simulink model "sl_pmsm"  (R2023b)
settings: Solver=VariableStepAuto  StartTime=0.0  StopTime=1.0  RelTol=1e-3
InitFcn:
  | init
values from neighbouring files (symbols this model uses):
  pa = block.DialogPrm(1).Data    [current_controller.m]    (also in voltage_equation_dq.m)
libraries: spsVoltageMeasurementLib x9, spsSeriesRLCBranchLib x3, simulink x3, spsDCVoltageSourceLib x2, slpidlib x1, spsGroundLib x1, spsUniversalBridgeLib x1, spspowerguiLib x1
settings Model: Creator=PC  LastModifiedBy=PC

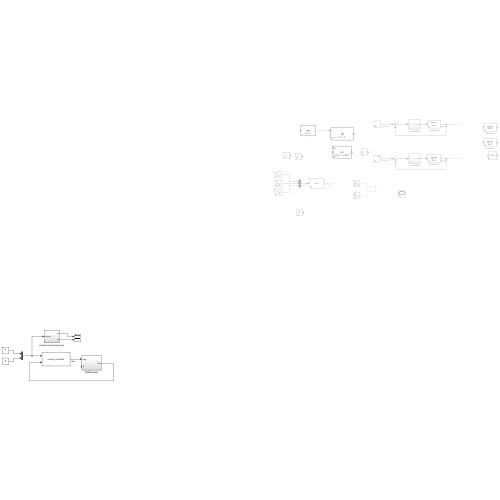
[thumbnail: Simulink's stored preview of the top-level diagram]
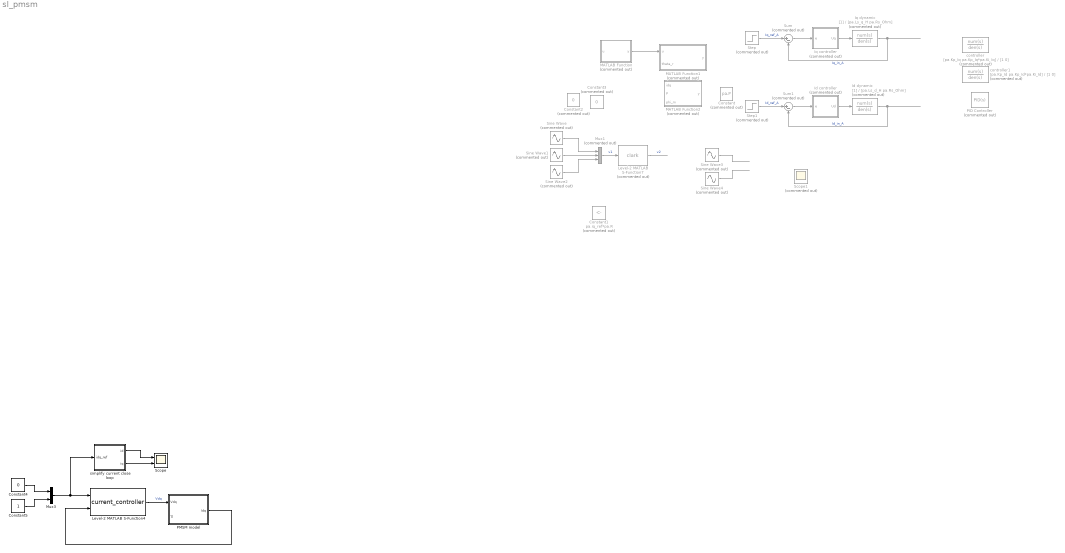
== system sl_pmsm ==
  Constant : Constant  Commented=on  Value=pa.P
  Constant1 : Constant  Commented=on  Value=pa.iq_ref*pa.R
  Constant2 : Constant  Commented=on  Value=0
  Constant3 : Constant  Commented=on  Value=0
  Constant4 : Constant  Value=0
  Constant5 : Constant
  Id controller : Subsystem  Commented=on
  Id dynamic : TransferFcn  Commented=on  Denominator=[pa.Ls_d_H pa.Rs_Ohm]
  Iq controller : Subsystem  Commented=on
  Iq dynamic : TransferFcn  Commented=on  Denominator=[pa.Ls_q_H pa.Rs_Ohm]
  Level-2 MATLAB S-Function4 : M-S-Function  FunctionName=current_controller  Parameters=pa
  Level-2 MATLAB S-Function7 : M-S-Function  Commented=on  FunctionName=clark  Parameters=pa
  MATLAB Function : MATLAB Function  Commented=on  TreatAsAtomicUnit=on
  MATLAB Function1 : MATLAB Function  Commented=on  TreatAsAtomicUnit=on
  MATLAB Function2 : MATLAB Function  Commented=on  TreatAsAtomicUnit=on
  Mux1 : Mux  Commented=on  Inputs=3
  Mux3 : Mux  Inputs=2
  PID Controller : slpidlib/PID Controller  Commented=on  Controller=PID  Form=Parallel  TimeDomain=Continuous-time  UseExternalTs=off  SampleTime=-1  IntegratorMethod=Forward Euler  FilterMethod=Forward Euler  ControllerParametersSource=internal  P=1  I=1  UseKiTs=off  D=0  N=100  UseFilter=on  TunerSelectOption=Transfer Function Based (PID Tuner App)  InitialConditionSource=internal  InitialConditionForIntegrator=0  InitialConditionForFilter=0  DifferentiatorICPrevScaledInput=0  ExternalReset=none  TrackingMode=off  Kt=1  LimitOutput=off  SatLimitsSource=internal  UpperSaturationLimit=inf  LowerSaturationLimit=-inf  LinearizeAsGain=on  AntiWindupMode=none  Kb=1  LimitIntegrator=off  UpperIntegratorSaturationLimit=inf  LowerIntegratorSaturationLimit=-inf  POutMin=[]  POutMax=[]  IOutMin=[]  IOutMax=[]  DOutMin=[]  DOutMax=[]  NOutMin=[]  NOutMax=[]  SumOutMin=[]  SumOutMax=[]  SaturationOutMin=[]  SaturationOutMax=[]  PParamMin=[]  PParamMax=[]  IParamMin=[]  IParamMax=[]  DParamMin=[]  DParamMax=[]  NParamMin=[]  NParamMax=[]  KbParamMin=[]  KbParamMax=[]  KtParamMin=[]  KtParamMax=[]  KbOutMin=[]  KbOutMax=[]  KtOutMin=[]  KtOutMax=[]  IntegratorOutMin=[]  IntegratorOutMax=[]  FilterOutMin=[]  FilterOutMax=[]  SumI1OutMin=[]  SumI1OutMax=[]  SumI2OutMin=[]  SumI2OutMax=[]  SumI3OutMin=[]  SumI3OutMax=[]  SumI4OutMin=[]  SumI4OutMax=[]  SumDOutMin=[]  SumDOutMax=[]  DifferentiatorOutMin=[]  DifferentiatorOutMax=[]  FilterDiffOutCoefMin=[]  FilterDiffOutCoefMax=[]  ReciprocalOutMin=[]  ReciprocalOutMax=[]  SumDenOutMin=[]  SumDenOutMax=[]  SumNumOutMin=[]  SumNumOutMax=[]  DivideOutMin=[]  DivideOutMax=[]  UdiffTsProdOutMin=[]  UdiffTsProdOutMax=[]  NTsProdOutMin=[]  NTsProdOutMax=[]  UintegralTsProdOutMin=[]  UintegralTsProdOutMax=[]  UngainTsProdOutMin=[]  UngainTsProdOutMax=[]  ClampingZeroOutDataTypeStr=Inherit: Inherit via back propagation  ClampingZeroOutMin=[]  ClampingZeroOutMax=[]  FilterDenConstantOutDataTypeStr=Inherit: Inherit via back propagation  FilterDenConstantOutMin=[]  FilterDenConstantOutMax=[]  PCopyOutDataTypeStr=Inherit: Inherit via back propagation  PCopyOutMin=[]  PCopyOutMax=[]  NCopyOutDataTypeStr=Inherit: Inherit via back propagation  NCopyOutMin=[]  NCopyOutMax=[]  IntegratorContinuousStateAttributes=''  IntegratorStateMustResolveToSignalObject=off  IntegratorRTWStateStorageClass=Auto  FilterContinuousStateAttributes=''  FilterStateMustResolveToSignalObject=off  FilterRTWStateStorageClass=Auto  ParallelPVariant=InternalParameters  IdealPVariant=Disabled  IVariant=InternalParameters  DVariant=InternalParameters  IntegratorVariant=Continuous  SatVariant=Disabled  AWVariant=Passthrough  PCopyVariant=Disabled  TRVariant=Disabled  FdbkBlocksVariant=Forward  IdealPFdbkVariant=Disabled  SatFdbkVariant=Disabled  DerivativeFilterVariant=ContFilter  NVariant=InternalParameters  NCopyVariant=Disabled  FilterICVariant=InternalICsFilter  IntegratorICVariant=InternalICs  ExternalResetVariant=Disabled  TRSumVariant=Passthrough  SumFdbkVariant=Disabled  SumVariant=Sum_PID  TsampFilterVariant=InternalTs  TsampNgainVariant=Passthrough  TsampIntegralVariant=Disabled_SignalSpec  ExternalSaturationOutDataTypeStr=Inherit: Same as second input
  PMSM model : Subsystem
  Scope : Scope  NumInputPorts=2
  Scope1 : Scope  Commented=on
  Sine Wave : Sin  Commented=on  Frequency=50*2*pi  SampleTime=0
  Sine Wave1 : Sin  Commented=on  Frequency=50*2*pi  Phase=-2*pi/3  SampleTime=0
  Sine Wave2 : Sin  Commented=on  Frequency=50*2*pi  Phase=2*pi/3  SampleTime=0
  Sine Wave3 : Sin  Commented=on  Frequency=50*2*pi  SampleTime=0
  Sine Wave4 : Sin  Commented=on  Frequency=50*2*pi  Phase=-pi/2  SampleTime=0
  Step : Step  Commented=on  SampleTime=0
  Step1 : Step  Commented=on  SampleTime=0
  Sum : Sum  Commented=on  Inputs=|+-
  Sum1 : Sum  Commented=on  Inputs=|+-
  controller : TransferFcn  Commented=on  Numerator=[pa.Kp_Iq pa.Kp_Iq*pa.Ki_Iq]  Denominator=[1 0]
  controller1 : TransferFcn  Commented=on  Numerator=[pa.Kp_Id pa.Kp_Id*pa.Ki_Id]  Denominator=[1 0]
  simplify current close loop : Subsystem
  wires:
  Iq dynamic/1 -> Sum/2  "Iq_in_A"
  Id dynamic/1 -> Sum1/2  "Id_in_A"
  Step/1 -> Sum/1  "Iq_ref_A"
  Id controller/1(Ud) -> Id dynamic/1
  Step1/1 -> Sum1/1  "Id_ref_A"
  Sum/1 -> Iq controller/1(e)
  Iq controller/1(Uq) -> Iq dynamic/1
  Sum1/1 -> Id controller/1(e)
  MATLAB Function/1(y) -> MATLAB Function1/1(u)
  Sine Wave/1 -> Mux1/1
  Sine Wave1/1 -> Mux1/2
  Sine Wave2/1 -> Mux1/3
  Mux1/1 -> Level-2 MATLAB S-Function7/1  "v1"
  Sine Wave3/1 -> ?
  Sine Wave4/1 -> ?
  Level-2 MATLAB S-Function7/1 -> ?  "v2"
  Constant4/1 -> Mux3/1
  Constant5/1 -> Mux3/2
  Mux3/1 -> simplify current close loop/1(idq_ref), Level-2 MATLAB S-Function4/1
  simplify current close loop/1(id) -> Scope/1
  simplify current close loop/2(iq) -> Scope/2
  Level-2 MATLAB S-Function4/1 -> PMSM model/1(Vdq)  "Vdq"
  PMSM model/1(Idq) -> Level-2 MATLAB S-Function4/2

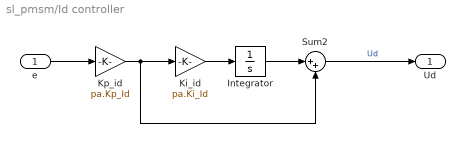
== system sl_pmsm/Id controller ==
  e : Inport
  Integrator : Integrator
  Ki_id : Gain  Gain=pa.Ki_Id
  Kp_id : Gain  Gain=pa.Kp_Id
  Sum2 : Sum  Inputs=|++
  Ud : Outport
  wires:
  Sum2/1 -> Ud/1  "Ud"
  Ki_id/1 -> Integrator/1
  e/1 -> Kp_id/1
  Kp_id/1 -> Ki_id/1, Sum2/2
  Integrator/1 -> Sum2/1

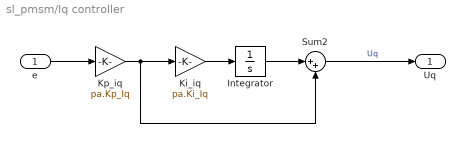
== system sl_pmsm/Iq controller ==
  e : Inport
  Integrator : Integrator
  Ki_iq : Gain  Gain=pa.Ki_Iq
  Kp_iq : Gain  Gain=pa.Kp_Iq
  Sum2 : Sum  Inputs=|++
  Uq : Outport
  wires:
  Integrator/1 -> Sum2/1
  Kp_iq/1 -> Sum2/2, Ki_iq/1
  e/1 -> Kp_iq/1
  Ki_iq/1 -> Integrator/1
  Sum2/1 -> Uq/1  "Uq"

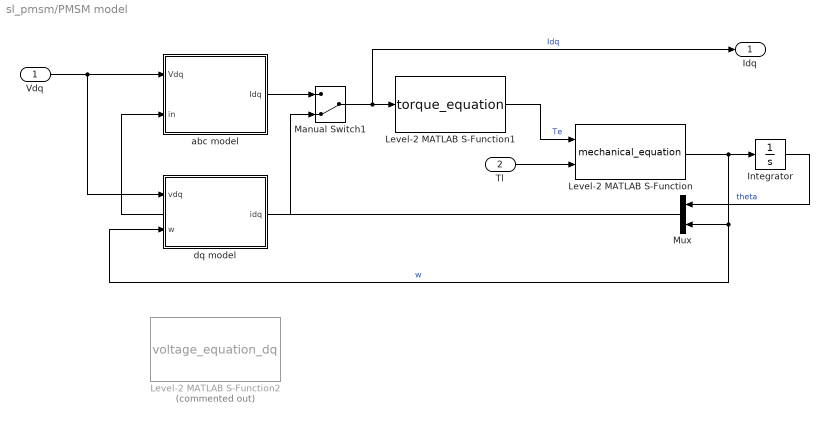
== system sl_pmsm/PMSM model ==
  Vdq : Inport
  Tl : Inport  Port=2
  Integrator : Integrator
  Level-2 MATLAB S-Function : M-S-Function  FunctionName=mechanical_equation  Parameters=pa
  Level-2 MATLAB S-Function1 : M-S-Function  FunctionName=torque_equation  Parameters=pa
  Level-2 MATLAB S-Function2 : M-S-Function  Commented=on  FunctionName=voltage_equation_dq  Parameters=pa
  Manual Switch1 : ManualSwitch  CurrentSetting=0
  Mux : Mux  Inputs=2
  abc model : Subsystem
  dq model : Subsystem
  Idq : Outport
  wires:
  Level-2 MATLAB S-Function1/1 -> Level-2 MATLAB S-Function/1  "Te"
  abc model/1(Idq) -> Manual Switch1/1
  Integrator/1 -> Mux/1  "theta"
  Level-2 MATLAB S-Function/1 -> dq model/2(w), Mux/2, Integrator/1  "w"
  Tl/1 -> Level-2 MATLAB S-Function/2
  dq model/1(idq) -> Manual Switch1/2
  Mux/1 -> abc model/2(in)
  Manual Switch1/1 -> Idq/1, Level-2 MATLAB S-Function1/1  "Idq"
  Vdq/1 -> dq model/1(vdq), abc model/1(Vdq)

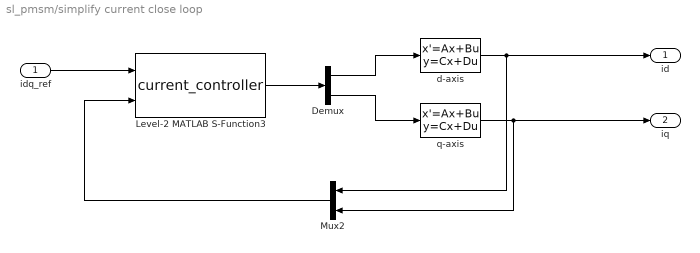
== system sl_pmsm/simplify current close loop ==
  idq_ref : Inport
  Demux : Demux  Outputs=2
  Level-2 MATLAB S-Function3 : M-S-Function  FunctionName=current_controller  Parameters=pa
  Mux2 : Mux  Inputs=2
  d-axis : StateSpace  A=-pa.R/pa.Ld  B=1/pa.Ld  D=0  InitialCondition=0
  q-axis : StateSpace  A=-pa.R/pa.Lq  B=1/pa.Lq  D=0  InitialCondition=0
  id : Outport
  iq : Outport  Port=2
  wires:
  Demux/2 -> q-axis/1
  d-axis/1 -> id/1, Mux2/1
  Mux2/1 -> Level-2 MATLAB S-Function3/2
  Level-2 MATLAB S-Function3/1 -> Demux/1
  q-axis/1 -> iq/1, Mux2/2
  Demux/1 -> d-axis/1
  idq_ref/1 -> Level-2 MATLAB S-Function3/1

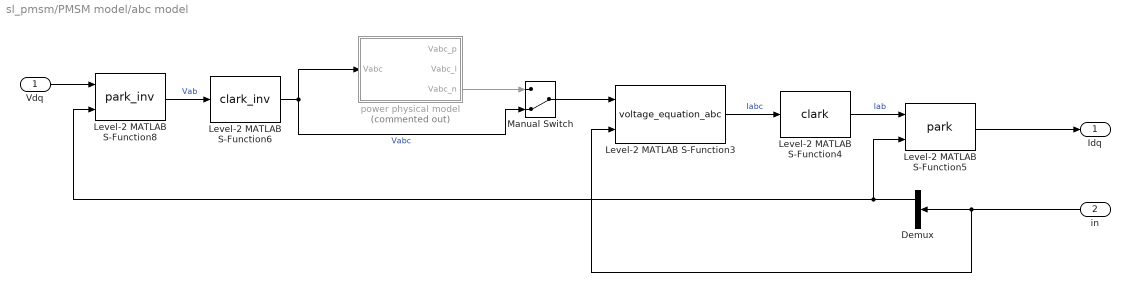
== system sl_pmsm/PMSM model/abc model ==
  Vdq : Inport
  in : Inport  Port=2
  Demux : Demux  Outputs=2
  Level-2 MATLAB S-Function3 : M-S-Function  FunctionName=voltage_equation_abc  Parameters=pa
  Level-2 MATLAB S-Function4 : M-S-Function  FunctionName=clark  Parameters=pa
  Level-2 MATLAB S-Function5 : M-S-Function  FunctionName=park  Parameters=pa
  Level-2 MATLAB S-Function6 : M-S-Function  FunctionName=clark_inv  Parameters=pa
  Level-2 MATLAB S-Function8 : M-S-Function  FunctionName=park_inv  Parameters=pa
  Manual Switch : ManualSwitch  CurrentSetting=0
  power physical model : Subsystem  Commented=on
  Idq : Outport
  wires:
  Level-2 MATLAB S-Function6/1 -> power physical model/1(Vabc), Manual Switch/2  "Vabc"
  Level-2 MATLAB S-Function8/1 -> Level-2 MATLAB S-Function6/1  "Vab"
  Level-2 MATLAB S-Function4/1 -> Level-2 MATLAB S-Function5/1  "Iab"
  Level-2 MATLAB S-Function3/1 -> Level-2 MATLAB S-Function4/1  "Iabc"
  Vdq/1 -> Level-2 MATLAB S-Function8/1
  Manual Switch/1 -> Level-2 MATLAB S-Function3/1
  power physical model/3(Vabc_n) -> Manual Switch/1
  Level-2 MATLAB S-Function5/1 -> Idq/1
  in/1 -> Level-2 MATLAB S-Function3/2, Demux/1
  Demux/1 -> Level-2 MATLAB S-Function8/2, Level-2 MATLAB S-Function5/2

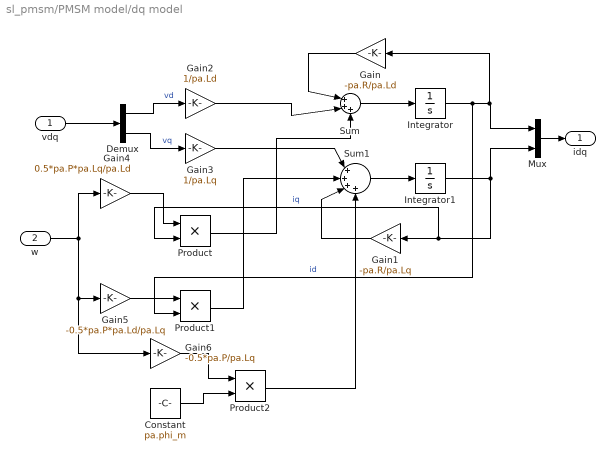
== system sl_pmsm/PMSM model/dq model ==
  vdq : Inport
  w : Inport  Port=2
  Constant : Constant  Value=pa.phi_m
  Demux : Demux  Outputs=2
  Gain : Gain  Gain=-pa.R/pa.Ld
  Gain1 : Gain  Gain=-pa.R/pa.Lq
  Gain2 : Gain  Gain=1/pa.Ld
  Gain3 : Gain  Gain=1/pa.Lq
  Gain4 : Gain  Gain=0.5*pa.P*pa.Lq/pa.Ld
  Gain5 : Gain  Gain=-0.5*pa.P*pa.Ld/pa.Lq
  Gain6 : Gain  Gain=-0.5*pa.P/pa.Lq
  Integrator : Integrator
  Integrator1 : Integrator
  Mux : Mux  Inputs=2
  Product : Product
  Product1 : Product
  Product2 : Product
  Sum : Sum  Inputs=|+++
  Sum1 : Sum  Inputs=|++++
  idq : Outport
  wires:
  Mux/1 -> idq/1
  Integrator/1 -> Product1/2, Gain/1, Mux/1  "id"
  Integrator1/1 -> Mux/2, Product/2, Gain1/1  "iq"
  vdq/1 -> Demux/1
  Sum/1 -> Integrator/1
  Sum1/1 -> Integrator1/1
  Gain/1 -> Sum/1
  Gain1/1 -> Sum1/3
  Demux/1 -> Gain2/1  "vd"
  Gain2/1 -> Sum/2
  Demux/2 -> Gain3/1  "vq"
  Gain3/1 -> Sum1/1
  w/1 -> Gain4/1, Gain6/1, Gain5/1
  Gain4/1 -> Product/1
  Product/1 -> Sum/3
  Gain5/1 -> Product1/1
  Product1/1 -> Sum1/2
  Gain6/1 -> Product2/1
  Constant/1 -> Product2/2
  Product2/1 -> Sum1/4

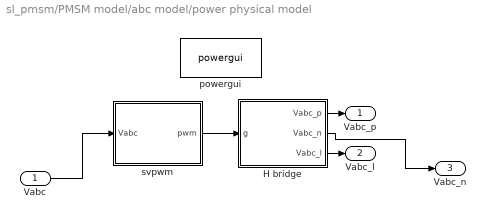
== system sl_pmsm/PMSM model/abc model/power physical model ==
  Vabc : Inport
  "H bridge " : Subsystem
  powergui : spspowerguiLib/powergui  Priority=1  SimulationMode=Continuous  SampleTime=50e-6  frequency=60  Iterations=50  frequencyindice=0  Pbase=100e6  ErrMax=1e-4  UnitsV=kV  UnitsW=MW  buscounter=0  FunctionMessages=off  echomessages=off  EnableUseOfTLC=off  CurrentSourceSwitches=off  DisableSnubberDevices=off  DisableRonSwitches=off  DisableVfSwitches=off  DisplayEquations=off  AutomaticDiscreteSolvers=off  SolverType=Tustin/Backward Euler (TBE)  Interpol=off  ExternalGateDelay=off  methode=off  Ts=100  x0status=blocks  SPID=on  SwTol=0  HookPort=off  NonlinearTolerance=1e-4  nMaxIteration=100  ContinueOnMaxIteration=off  RestoreLinks=warning  ResistiveCurrentMeasurement=off  Frange=[0:2:500]  Ylog=off  Xlog=on  ShowGrid=off  save=off  variable=ZData  structure=0  ZoomFFT=off  StartTime=0.0  cycles=1  DisplayStyle=1  fundamental=60  FreqAxis=off  MaxFrequency=1000  frequencyindicesteady=1  RmsSteady=1  display=off
  svpwm : Subsystem
  Vabc_p : Outport
  Vabc_l : Outport  Port=2
  Vabc_n : Outport  Port=3
  wires:
  svpwm/1(pwm) -> "H bridge "/1(g)
  "H bridge "/2(Vabc_n) -> Vabc_n/1
  "H bridge "/1(Vabc_p) -> Vabc_p/1
  Vabc/1 -> svpwm/1(Vabc)
  "H bridge "/3(Vabc_l) -> Vabc_l/1

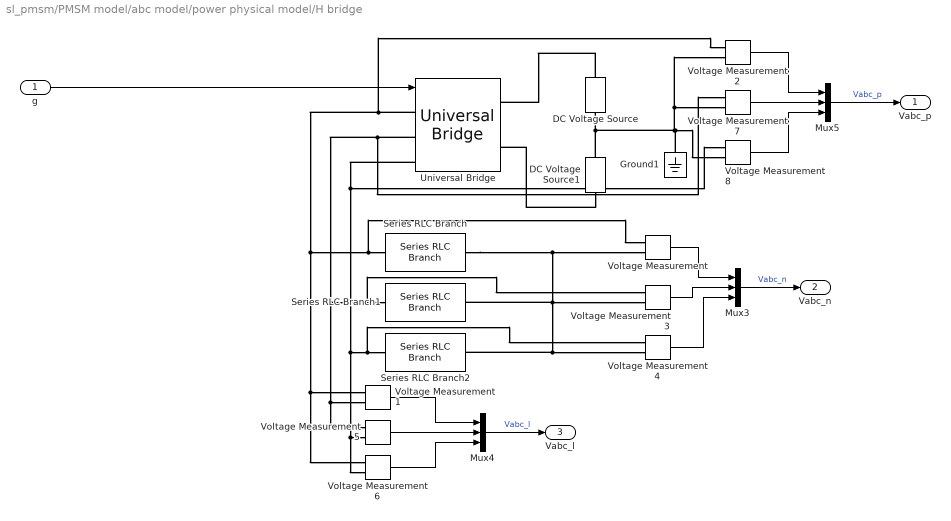
== system sl_pmsm/PMSM model/abc model/power physical model/H bridge  ==
  g : Inport
  DC Voltage Source : spsDCVoltageSourceLib/DC Voltage Source  Amplitude=pa.dc/2  Measurements=None
  DC Voltage Source1 : spsDCVoltageSourceLib/DC Voltage Source  Amplitude=pa.dc/2  Measurements=None
  Ground1 : spsGroundLib/Ground  LConnTagsString=a
  Mux3 : Mux  Inputs=3
  Mux4 : Mux  Inputs=3
  Mux5 : Mux  Inputs=3
  Series RLC Branch : spsSeriesRLCBranchLib/Series RLC Branch  LConnTagsString=__new0  RConnTagsString=__new0  BranchType=RL  Resistance=1  Inductance=1e-3  SetiL0=off  InitialCurrent=0  Capacitance=1e-6  Setx0=off  InitialVoltage=0  Measurements=None
  Series RLC Branch1 : spsSeriesRLCBranchLib/Series RLC Branch  LConnTagsString=__new0  RConnTagsString=__new0  BranchType=RL  Resistance=1  Inductance=1e-3  SetiL0=off  InitialCurrent=0  Capacitance=1e-6  Setx0=off  InitialVoltage=0  Measurements=None
  Series RLC Branch2 : spsSeriesRLCBranchLib/Series RLC Branch  LConnTagsString=__new0  RConnTagsString=__new0  BranchType=RL  Resistance=1  Inductance=1e-3  SetiL0=off  InitialCurrent=0  Capacitance=1e-6  Setx0=off  InitialVoltage=0  Measurements=None
  Universal Bridge : spsUniversalBridgeLib/Universal Bridge  Arms=3  SnubberResistance=1e5  SnubberCapacitance=inf  Device=MOSFET / Diodes  Ron=1e-3  Lon=0  ForwardVoltages="[  0  0  ]"  ForwardVoltage=0  GTOparameters=[ 10e-6 , 20e-6 ]  IGBTparameters=[ 1e-6 , 2e-6 ]  Measurements=None  Measurements_2=None  converterType=Rectifier
  Voltage Measurement{,1..8} (9 alike) : spsVoltageMeasurementLib/Voltage Measurement  PhasorSimulation=off  OutputType=Complex  PSBequivalent=0
  Vabc_p : Outport
  Vabc_n : Outport  Port=2
  Vabc_l : Outport  Port=3
  wires:
  Voltage Measurement2/1 -> Mux5/1
  Voltage Measurement1/1 -> Mux4/1
  Voltage Measurement/1 -> Mux3/1
  Voltage Measurement6/1 -> Mux4/3
  Voltage Measurement3/1 -> Mux3/2
  Voltage Measurement8/1 -> Mux5/3
  Voltage Measurement4/1 -> Mux3/3
  Voltage Measurement7/1 -> Mux5/2
  Voltage Measurement5/1 -> Mux4/2
  Mux5/1 -> Vabc_p/1  "Vabc_p"
  Mux4/1 -> Vabc_l/1  "Vabc_l"
  Mux3/1 -> Vabc_n/1  "Vabc_n"
  g/1 -> Universal Bridge/1
  connections:
  Universal Bridge/LConn3 -- Voltage Measurement8/LConn1 -- Voltage Measurement6/LConn2 -- Voltage Measurement5/LConn2 -- Voltage Measurement4/LConn1 -- Series RLC Branch2/LConn1
  Universal Bridge/LConn1 -- Voltage Measurement2/LConn1 -- Voltage Measurement6/LConn1 -- Voltage Measurement1/LConn1 -- Voltage Measurement/LConn1 -- Series RLC Branch/LConn1
  Universal Bridge/LConn2 -- Voltage Measurement7/LConn1 -- Voltage Measurement1/LConn2 -- Voltage Measurement5/LConn1 -- Voltage Measurement3/LConn1 -- Series RLC Branch1/LConn1
  DC Voltage Source1/RConn1 -- Ground1/LConn1 -- Voltage Measurement8/LConn2 -- Voltage Measurement7/LConn2 -- Voltage Measurement2/LConn2 -- DC Voltage Source/LConn1
  DC Voltage Source/RConn1 -- Universal Bridge/RConn1
  DC Voltage Source1/LConn1 -- Universal Bridge/RConn2
  Series RLC Branch/RConn1 -- Voltage Measurement3/LConn2 -- Series RLC Branch1/RConn1 -- Series RLC Branch2/RConn1 -- Voltage Measurement4/LConn2 -- Voltage Measurement/LConn2

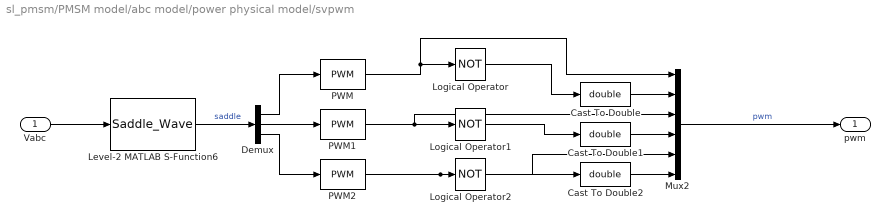
== system sl_pmsm/PMSM model/abc model/power physical model/svpwm ==
  Vabc : Inport
  Cast To Double : DataTypeConversion  OutDataTypeStr=double  SaturateOnIntegerOverflow=off  RndMeth=Floor
  Cast To Double1 : DataTypeConversion  OutDataTypeStr=double  SaturateOnIntegerOverflow=off  RndMeth=Floor
  Cast To Double2 : DataTypeConversion  OutDataTypeStr=double  SaturateOnIntegerOverflow=off  RndMeth=Floor
  Demux : Demux  Outputs=3
  Level-2 MATLAB S-Function6 : M-S-Function  FunctionName=Saddle_Wave  Parameters=pa
  Logical Operator : Logic  Operator=NOT  AllPortsSameDT=off  OutDataTypeStr=boolean
  Logical Operator1 : Logic  Operator=NOT  AllPortsSameDT=off  OutDataTypeStr=boolean
  Logical Operator2 : Logic  Operator=NOT  AllPortsSameDT=off  OutDataTypeStr=boolean
  Mux2 : Mux  Inputs=6
  PWM : simulink/Discontinuities/PWM  DisableCoverage=on  Period=1/(pa.CarrFreq*1000)  InitialDelay=0  DisallowZeroDutyCycle=off  RunAtFixedTimeIntervals=off  SampleTime=0.1
  PWM1 : simulink/Discontinuities/PWM  DisableCoverage=on  Period=1/(pa.CarrFreq*1000)  InitialDelay=0  DisallowZeroDutyCycle=off  RunAtFixedTimeIntervals=off  SampleTime=0.1
  PWM2 : simulink/Discontinuities/PWM  DisableCoverage=on  Period=1/(pa.CarrFreq*1000)  InitialDelay=0  DisallowZeroDutyCycle=off  RunAtFixedTimeIntervals=off  SampleTime=0.1
  pwm : Outport
  wires:
  PWM1/1 -> Logical Operator1/1, Mux2/3
  Logical Operator/1 -> Cast To Double/1
  Mux2/1 -> pwm/1  "pwm"
  Vabc/1 -> Level-2 MATLAB S-Function6/1
  PWM/1 -> Mux2/1, Logical Operator/1
  Logical Operator2/1 -> Cast To Double2/1
  Demux/2 -> PWM1/1
  Demux/1 -> PWM/1
  Cast To Double2/1 -> Mux2/6
  PWM2/1 -> Mux2/5, Logical Operator2/1
  Level-2 MATLAB S-Function6/1 -> Demux/1  "saddle"
  Cast To Double/1 -> Mux2/2
  Logical Operator1/1 -> Cast To Double1/1
  Demux/3 -> PWM2/1
  Cast To Double1/1 -> Mux2/4

== matlab function sl_pmsm/MATLAB Function1 ==
  data: u input; y output; theta_r input; pa data_store_memory
function y = park_tf(u,theta_r)
global pa;
P = pa.P;
theta_e = P/2 * theta_r;
park = [cos(theta_e) sin(theta_e);
        -sin(theta_e) cos(theta_e)];
y = park*u;

== matlab function sl_pmsm/MATLAB Function ==
  data: u input; y output
function y = clark_tf(u)
clark = 2/3 * [1 -1/2 -1/2;
               0 sqrt(3)/2 -sqrt(3)/2];
y = clark*u;

== matlab function sl_pmsm/MATLAB Function2 ==
  data: idq input; y output; P input; phi_m input
function y = torque_equation(idq,P,phi_m)

ied = idq(1);
ieq = idq(2);

phi_m = pa.phi_m;
P = pa.P;

% Te = 3*P/4 *(phi_m*ieq - (Lq-Ld)*ied*ieq);
Te = 3*P/4 *(phi_m*ieq);

y = Te;
